simulink model "Home_exam_retake_sim"  (R2023a)
settings: Solver=FixedStepAuto  StartTime=0.0  StopTime=10.0  FixedStep=0.001  RelTol=1e-3
model workspace (MAT data in the model file):
  StepTime = 1
values from neighbouring files (symbols this model uses):
  A_m = 0    [home_exam_retake.m]
  B_m = 0    [home_exam_retake.m]
  Bt = Bt_array(test)    [home_exam_retake.m]
  C_m = 0    [home_exam_retake.m]
  const = 0    [home_exam_retake.m]
  D_m = 0    [home_exam_retake.m]
  denum = [a]    [home_exam_retake.m]
  Ks = Ks_array(test)    [home_exam_retake.m]
  Kt = Kt_array(test)    [home_exam_retake.m]
  Msprung = Msprung_array(test)    [home_exam_retake.m]
  Munsprung = Munsprung_array(test)    [home_exam_retake.m]
  numm = [b]    [home_exam_retake.m]
  ramp_slope = ramp_slopes(scenario)    [home_exam_retake.m]
  step2_fvalue = step2_final_values(scenario)    [home_exam_retake.m]
  step_stime = step_time(scenario)    [home_exam_retake.m]
libraries: simulink x1
settings Model: Creator=samer  LastModifiedBy=samer

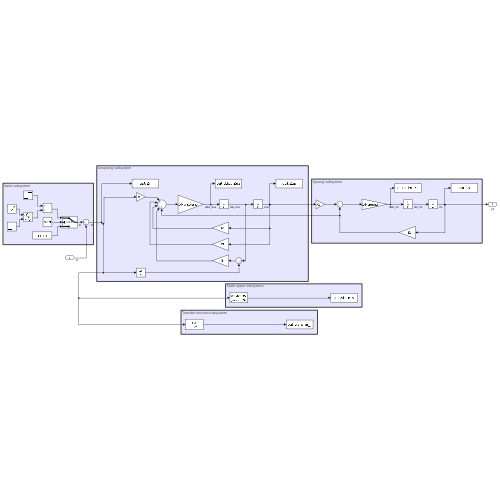
[thumbnail: Simulink's stored preview of the top-level diagram]
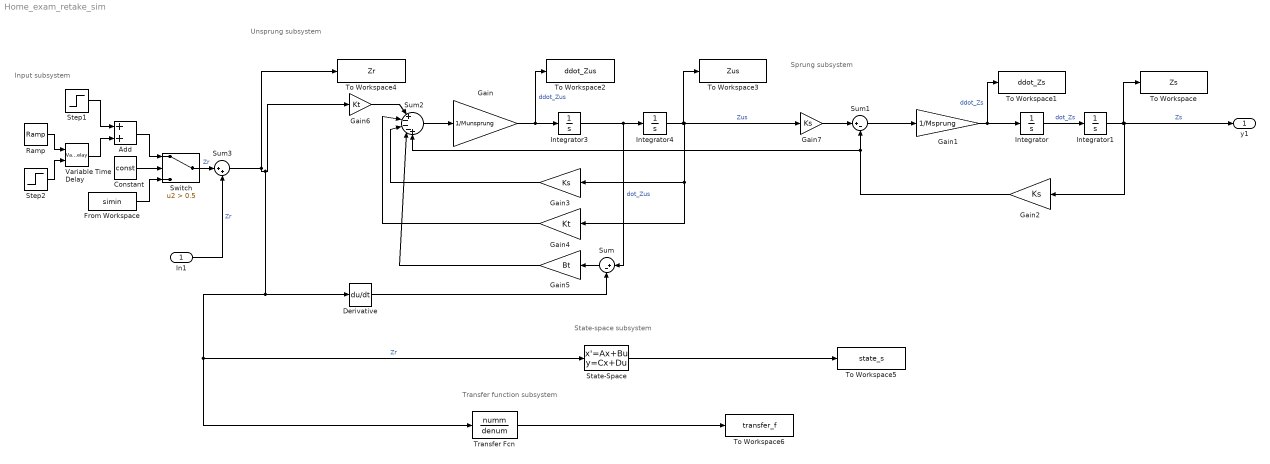
== system Home_exam_retake_sim ==
  note: Transfer function subsystem
  note: State-space subsystem
  note: Input subsystem
  note: Sprung subsystem
  note: Unsprung subsystem
  In1 : Inport
  Add : Sum
  Constant : Constant  Value=const
  Derivative : Derivative
  From Workspace : FromWorkspace  VariableName=simin  OutDataTypeStr=double
  Gain : Gain  Gain=1/Munsprung
  Gain1 : Gain  Gain=1/Msprung
  Gain2 : Gain  Gain=Ks
  Gain3 : Gain  Gain=Ks
  Gain4 : Gain  Gain=Kt
  Gain5 : Gain  Gain=Bt
  Gain6 : Gain  Gain=Kt
  Gain7 : Gain  Gain=Ks
  Integrator{,1,3..4} (4 alike) : Integrator
  Ramp : simulink/Sources/Ramp  slope=ramp_slope  start=ramp_stime  InitialOutput=0
  State-Space : StateSpace  A=A_m  B=B_m  C=C_m  D=D_m  InitialCondition=0
  Step1 : Step  Time=step_stime  After=0.005  SampleTime=0
  Step2 : Step  Time=step_stime  After=step2_fvalue  SampleTime=0
  Sum : Sum  Inputs=|+-
  Sum1 : Sum  Inputs=|+-
  Sum2 : Sum  Inputs=|+---+
  Sum3 : Sum  Inputs=|++
  Switch : Switch  Criteria=u2 > Threshold  Threshold=0.5  SaturateOnIntegerOverflow=off  InputSameDT=off
  To Workspace : ToWorkspace  VariableName=Zs  SampleTime=-1
  To Workspace1 : ToWorkspace  VariableName=ddot_Zs  SampleTime=-1
  To Workspace2 : ToWorkspace  VariableName=ddot_Zus  SampleTime=-1
  To Workspace3 : ToWorkspace  VariableName=Zus  SampleTime=-1
  To Workspace4 : ToWorkspace  VariableName=Zr  SampleTime=-1
  To Workspace5 : ToWorkspace  VariableName=state_s  SampleTime=-1
  To Workspace6 : ToWorkspace  VariableName=transfer_f  SampleTime=-1
  Transfer Fcn : TransferFcn  Numerator=numm  Denominator=denum
  Variable Time Delay : VariableTransportDelay  MaximumDelay=10
  y1 : Outport
  wires:
  Integrator3/1 -> Sum/1, Integrator4/1  "dot_Zus"
  Gain4/1 -> Sum2/2
  Integrator4/1 -> Gain7/1, Gain4/1, Gain3/1, To Workspace3/1  "Zus"
  Derivative/1 -> Sum/2
  Gain/1 -> To Workspace2/1, Integrator3/1  "ddot_Zus"
  Gain3/1 -> Sum2/3
  Gain5/1 -> Sum2/4
  Sum2/1 -> Gain/1
  Gain6/1 -> Sum2/1
  Gain2/1 -> Sum1/2, Sum2/5
  Sum/1 -> Gain5/1
  In1/1 -> Sum3/2  "Zr"
  Gain1/1 -> To Workspace1/1, Integrator/1  "ddot_Zs"
  Integrator1/1 -> y1/1, Gain2/1, To Workspace/1  "Zs"
  Gain7/1 -> Sum1/1
  Sum1/1 -> Gain1/1
  Integrator/1 -> Integrator1/1  "dot_Zs"
  Sum3/1 -> Transfer Fcn/1, State-Space/1, Derivative/1, Gain6/1, To Workspace4/1  "Zr"
  Step1/1 -> Add/1
  Variable Time Delay/1 -> Add/2
  Step2/1 -> Variable Time Delay/2
  Add/1 -> Switch/1
  Switch/1 -> Sum3/1  "Zr"
  From Workspace/1 -> Switch/3
  Constant/1 -> Switch/2
  Ramp/1 -> Variable Time Delay/1
  State-Space/1 -> To Workspace5/1
  Transfer Fcn/1 -> To Workspace6/1
